simulink model "Quaternion_TestModel"  (R2014a)
settings: Solver=ode45  StartTime=0.0  StopTime=10.0  RelTol=1e-3
libraries: aerolib6dof2 x1
settings Model: Creator=scorpii  LastModifiedBy=scorpii

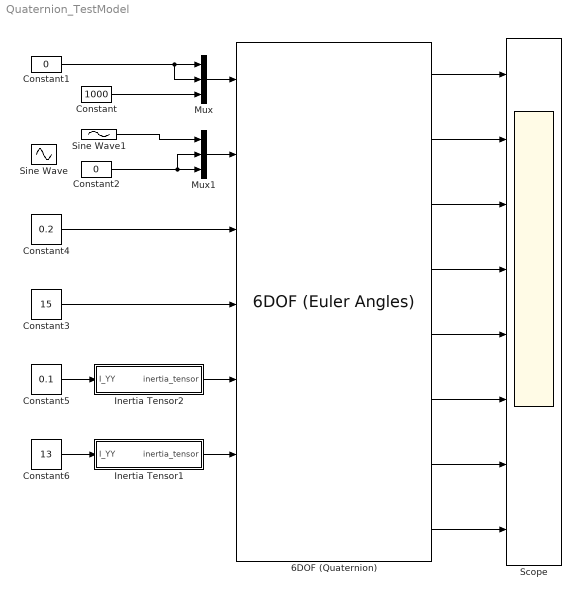
== system Quaternion_TestModel ==
  6DOF (Quaternion) : aerolib6dof2/6DOF (Euler Angles)  units=Metric (MKS)  mtype=Custom Variable  rep=Quaternion  xme_0=[0 0 0]  Vm_0=[0 0 0]  eul_0=[0 0 0]  pm_0=[0 0 0]  mass_0=1.0  mass_e=0.5  mass_f=2.0  inertia=eye(3)  inertia_e=eye(3)  inertia_f=2*eye(3)  k_quat=1.0  vre_flag=on
  Constant : Constant  Value=1000
  Constant1 : Constant  Value=0
  Constant2 : Constant  Value=0
  Constant3 : Constant  Value=15
  Constant4 : Constant  Value=0.2
  Constant5 : Constant  Value=0.1
  Constant6 : Constant  Value=13
  Inertia Tensor1 : Subsystem
  Inertia Tensor2 : Subsystem
  Mux : Mux  Inputs=3
  Mux1 : Mux  Inputs=3
  Scope : Scope  NumInputPorts=8
      settings: TimeRange=1  YMin=0~0~0~0~0~0~0~0  YMax=1~1~1~1~1~1~1~1
  Sine Wave : Sin  SampleTime=0
  Sine Wave1 : Sin  Amplitude=10  SampleTime=0
  wires:
  6DOF (Quaternion)/6 -> Scope/6
  6DOF (Quaternion)/3 -> Scope/3
  6DOF (Quaternion)/2 -> Scope/2
  6DOF (Quaternion)/1 -> Scope/1
  6DOF (Quaternion)/5 -> Scope/5
  6DOF (Quaternion)/4 -> Scope/4
  6DOF (Quaternion)/7 -> Scope/7
  6DOF (Quaternion)/8 -> Scope/8
  Mux/1 -> 6DOF (Quaternion)/1
  Constant/1 -> Mux/3
  Constant1/1 -> Mux/2, Mux/1
  Mux1/1 -> 6DOF (Quaternion)/2
  Constant2/1 -> Mux1/2, Mux1/3
  Constant4/1 -> 6DOF (Quaternion)/3
  Constant3/1 -> 6DOF (Quaternion)/4
  Constant5/1 -> Inertia Tensor2/1(I_YY)
  Inertia Tensor1/1(inertia_tensor) -> 6DOF (Quaternion)/6
  Constant6/1 -> Inertia Tensor1/1(I_YY)
  Inertia Tensor2/1(inertia_tensor) -> 6DOF (Quaternion)/5
  Sine Wave1/1 -> Mux1/1

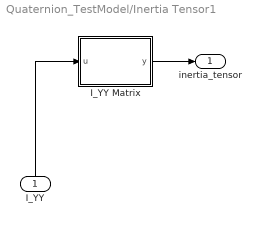
== system Quaternion_TestModel/Inertia Tensor1 ==
  I_YY : Inport
  I_YY Matrix : MATLAB Function  TreatAsAtomicUnit=on
  inertia_tensor : Outport
  wires:
  I_YY Matrix/1(y) -> inertia_tensor/1
  I_YY/1 -> I_YY Matrix/1(u)

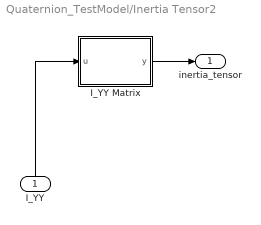
== system Quaternion_TestModel/Inertia Tensor2 ==
  I_YY : Inport
  I_YY Matrix : MATLAB Function  TreatAsAtomicUnit=on
  inertia_tensor : Outport
  wires:
  I_YY Matrix/1(y) -> inertia_tensor/1
  I_YY/1 -> I_YY Matrix/1(u)

== matlab function Quaternion_TestModel/Inertia Tensor1/I_YY Matrix ==
  data: u input; y output
function y = fcn(u)
y = [ u 0 0; 0 0 0; 0 0 0 ];

== matlab function Quaternion_TestModel/Inertia Tensor2/I_YY Matrix ==
  data: u input; y output
function y = fcn(u)
y = [ u 0 0; 0 0 0; 0 0 0 ];
